simulink subsystem "Robot_sub"  (R2023b)
settings: Solver=VariableStepAuto  StartTime=0.0  StopTime=10.0  RelTol=1e-3
undefined symbols (not defined in the file): Frequency, Offset, t_sample
settings Model: Creator=ander  LastModifiedBy=ander

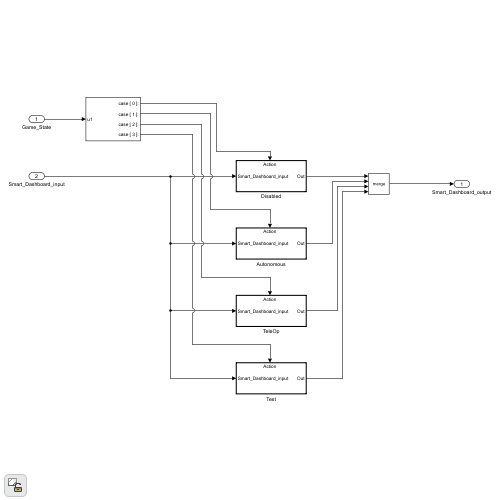
[thumbnail: Simulink's stored preview of the top-level diagram]
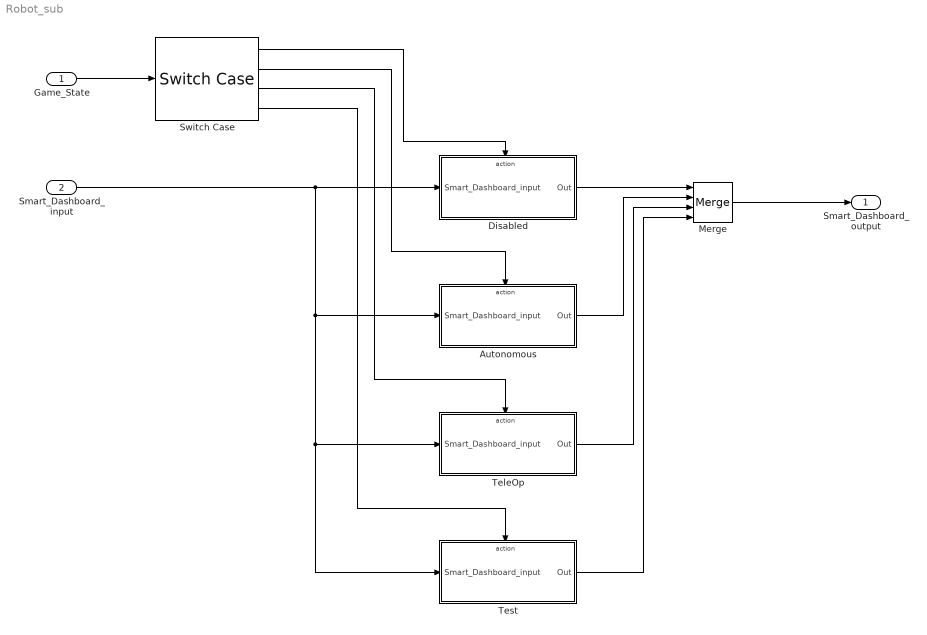
== system Robot_sub ==
  Game_State : Inport
  Smart_Dashboard_input : Inport  Port=2
  Autonomous : Subsystem  TreatAsAtomicUnit=on
  Disabled : Subsystem  TreatAsAtomicUnit=on
  Merge : Merge  Inputs=4
  Switch Case : SwitchCase  CaseConditions={0,1,2,3}  ShowDefaultCase=off
  TeleOp : Subsystem  TreatAsAtomicUnit=on
  Test : Subsystem  TreatAsAtomicUnit=on
  Smart_Dashboard_output : Outport
  wires:
  TeleOp/1(Out) -> Merge/3
  Autonomous/1(Out) -> Merge/2
  Disabled/1(Out) -> Merge/1
  Smart_Dashboard_input/1 -> Disabled/1(Smart_Dashboard_input), TeleOp/1(Smart_Dashboard_input), Test/1(Smart_Dashboard_input), Autonomous/1(Smart_Dashboard_input)
  Game_State/1 -> Switch Case/1
  Switch Case/1 -> Disabled/Action
  Switch Case/3 -> TeleOp/Action
  Switch Case/4 -> Test/Action
  Test/1(Out) -> Merge/4
  Merge/1 -> Smart_Dashboard_output/1
  Switch Case/2 -> Autonomous/Action

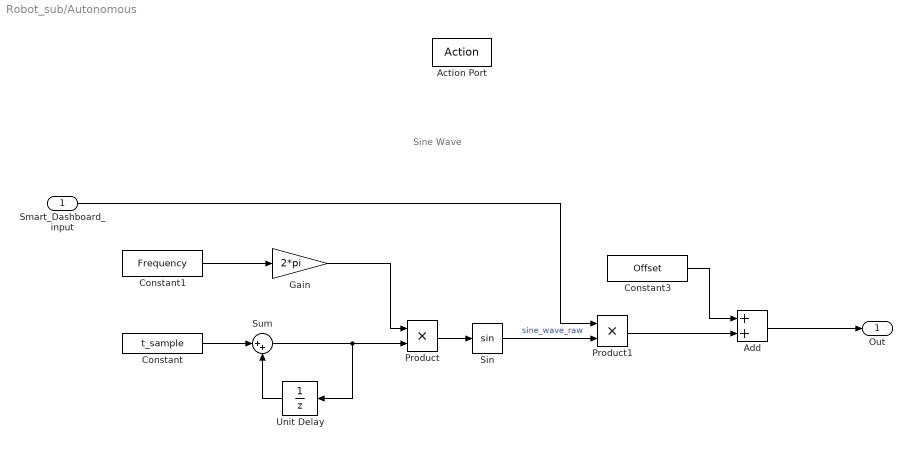
== system Robot_sub/Autonomous ==
  note: Sine Wave
  Smart_Dashboard_input : Inport
  Action Port : ActionPort  InitializeStates=reset
  Add : Sum
  Constant : Constant  Value=t_sample
  Constant1 : Constant  Value=Frequency
  Constant3 : Constant  Value=Offset
  Gain : Gain  Gain=2*pi
  Product : Product
  Product1 : Product
  Sin : Trigonometry
  Sum : Sum  Inputs=|++
  Unit Delay : UnitDelay  SampleTime=-1  HasFrameUpgradeWarning=on
  Out : Outport
  wires:
  Gain/1 -> Product/1
  Smart_Dashboard_input/1 -> Product1/1
  Product1/1 -> Add/2
  Unit Delay/1 -> Sum/2
  Sin/1 -> Product1/2  "sine_wave_raw"
  Add/1 -> Out/1
  Constant3/1 -> Add/1
  Constant1/1 -> Gain/1
  Product/1 -> Sin/1
  Sum/1 -> Unit Delay/1, Product/2
  Constant/1 -> Sum/1

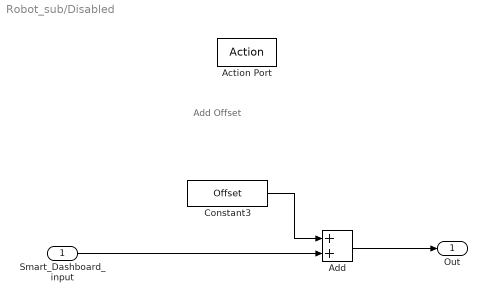
== system Robot_sub/Disabled ==
  note: Add Offset
  Smart_Dashboard_input : Inport
  Action Port : ActionPort
  Add : Sum
  Constant3 : Constant  Value=Offset
  Out : Outport
  wires:
  Add/1 -> Out/1
  Smart_Dashboard_input/1 -> Add/2
  Constant3/1 -> Add/1

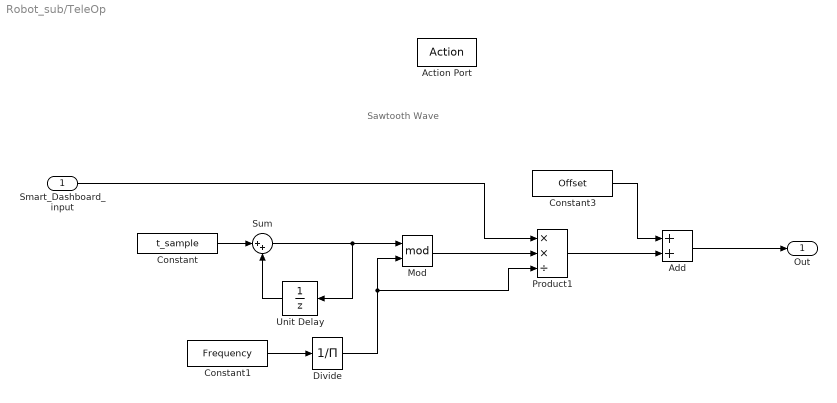
== system Robot_sub/TeleOp ==
  note: Sawtooth Wave
  Smart_Dashboard_input : Inport
  Action Port : ActionPort  InitializeStates=reset
  Add : Sum
  Constant : Constant  Value=t_sample
  Constant1 : Constant  Value=Frequency
  Constant3 : Constant  Value=Offset
  Divide : Product  Inputs=/
  Mod : Math  Operator=mod
  Product1 : Product  Inputs=**/
  Sum : Sum  Inputs=|++
  Unit Delay : UnitDelay  SampleTime=-1  HasFrameUpgradeWarning=on
  Out : Outport
  wires:
  Mod/1 -> Product1/2
  Constant/1 -> Sum/1
  Sum/1 -> Unit Delay/1, Mod/1
  Divide/1 -> Mod/2, Product1/3
  Constant1/1 -> Divide/1
  Unit Delay/1 -> Sum/2
  Smart_Dashboard_input/1 -> Product1/1
  Product1/1 -> Add/2
  Add/1 -> Out/1
  Constant3/1 -> Add/1

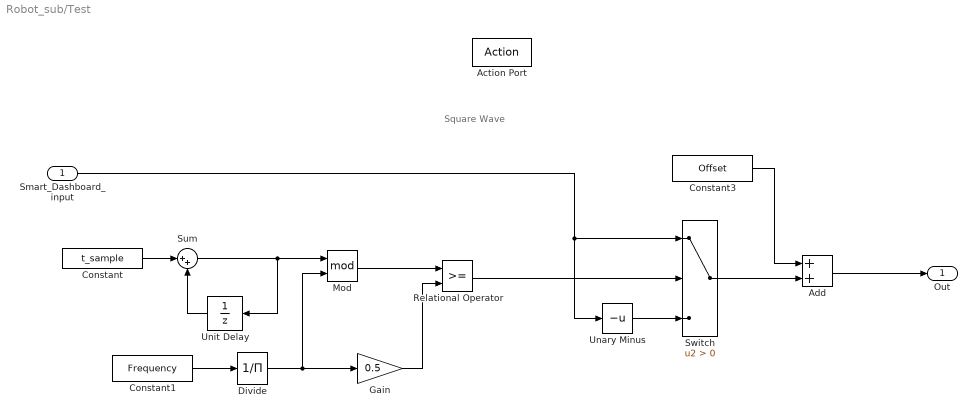
== system Robot_sub/Test ==
  note: Square Wave
  Smart_Dashboard_input : Inport
  Action Port : ActionPort  InitializeStates=reset
  Add : Sum
  Constant : Constant  Value=t_sample
  Constant1 : Constant  Value=Frequency
  Constant3 : Constant  Value=Offset
  Divide : Product  Inputs=/
  Gain : Gain  Gain=0.5
  Mod : Math  Operator=mod
  Relational Operator : RelationalOperator  OutDataTypeStr=boolean  RndMeth=Simplest  InputSameDT=off
  Sum : Sum  Inputs=|++
  Switch : Switch  Criteria=u2 > Threshold  SaturateOnIntegerOverflow=off  InputSameDT=off
  Unary Minus : UnaryMinus
  Unit Delay : UnitDelay  SampleTime=-1  HasFrameUpgradeWarning=on
  Out : Outport
  wires:
  Unary Minus/1 -> Switch/3
  Smart_Dashboard_input/1 -> Switch/1, Unary Minus/1
  Switch/1 -> Add/2
  Unit Delay/1 -> Sum/2
  Sum/1 -> Unit Delay/1, Mod/1
  Constant/1 -> Sum/1
  Constant1/1 -> Divide/1
  Divide/1 -> Mod/2, Gain/1
  Gain/1 -> Relational Operator/2
  Mod/1 -> Relational Operator/1
  Relational Operator/1 -> Switch/2
  Add/1 -> Out/1
  Constant3/1 -> Add/1
